simulink model "Eg5_4"  (R2018a)
settings: Solver=VariableStepAuto  StartTime=0.0  StopTime=10.0  RelTol=1e-3
settings Model: Creator=wangluo  LastModifiedBy=wangluo

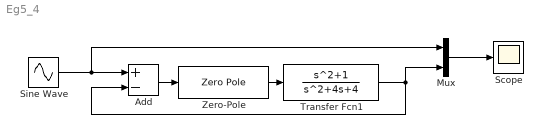
== system Eg5_4 ==
  Add : Sum  Inputs=+-
  Mux : Mux  Inputs=2
  Scope : Scope
  Sine Wave : Sin  SampleTime=0
  Transfer Fcn1 : TransferFcn  Numerator=[1 0 1]  Denominator=[1 4 4]
  Zero-Pole : ZeroPole  Zeros=[-5]  Poles=[-1 -3]
  wires:
  Add/1 -> Zero-Pole/1
  Zero-Pole/1 -> Transfer Fcn1/1
  Mux/1 -> Scope/1
  Transfer Fcn1/1 -> Add/2, Mux/2
  Sine Wave/1 -> Mux/1, Add/1
